simulink model "Model_tank"  (R2021b)
settings: Solver=ode45  StartTime=0.0  StopTime=80  RelTol=1e-3  EnableMultiTasking=on
values from neighbouring files (symbols this model uses):
  alpha1 = x1_val(2)    [Zbiorniki.m]    (also in c_table.mat = 0.278702458398; x0_table.mat = 0.278702458398)
  alpha2 = x2_val(2)    [Zbiorniki.m]    (also in c_table.mat = 0.328939614245; x0_table.mat = 0.328939614245)
  alpha3 = x3_val(2)    [Zbiorniki.m]    (also in c_table.mat = 0.404471667446; x0_table.mat = 0.404471667446)
  c1 = x1_val(1)    [Zbiorniki.m]    (also in c_table.mat = 41.0862215805; parametry.mat = 44.608; x0_table.mat = 41.0862215805)
  c2 = x2_val(1)    [Zbiorniki.m]    (also in c_table.mat = 36.7397635112; parametry.mat = 38.7996; x0_table.mat = 36.7397635112)
  c3 = x3_val(1)    [Zbiorniki.m]    (also in c_table.mat = 25.9394235455; parametry.mat = 39.9059; x0_table.mat = 25.9394235455)
undefined symbols (not defined in the file or in its folder): Set_Value_Motor
settings Model: Creator=Student  LastModifiedBy=Dawid
settings SolverCC: AlgebraicLoopSolver=TrustRegion
settings DataIOCC: LimitDataPoints=on  SaveFormat=Array  ReturnWorkspaceOutputs=off
settings OptimizationCC: LifeSpan=inf
settings DebuggingCC: SFUnexpectedBacktrackingDiag=warning  SFNoUnconditionalDefaultTransitionDiag=warning  SFExecutionAtInitializationDiag=none  SFMachineParentedDataDiag=warning  ArithmeticOperatorsInVariantConditions=warning
settings HardwareCC: ProdBitPerPointer=32  ProdBitPerSizeT=32  ProdBitPerPtrDiffT=32  ProdLargestAtomicFloat=None  ProdIntDivRoundTo=Undefined  ProdEndianess=Unspecified  ProdWordSize=32  ProdHWDeviceType=32-bit Generic
settings ModelReferenceCC: PropagateSignalLabelsOutOfModel=off
settings SFSimCC: SimUseLocalCustomCode=off  CustomCodeUndefinedFunction=UseInterfaceOnly
settings RTWCC: RTWUseLocalCustomCode=off
settings CodeAppCC: StateflowObjectComments=on
settings GRTTargetCC: TargetLangStandard=C89/C90 (ANSI)
settings ConfigComp: CovMetricSettings=dw  CovSaveCumulativeToWorkspaceVar=on  CovSaveSingleToWorkspaceVar=on  CovExternalEMLEnable=off

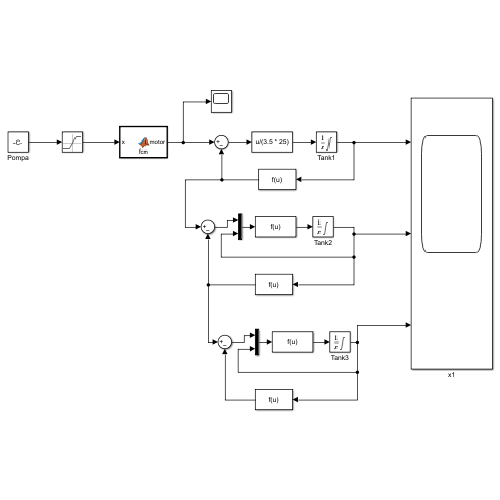
[thumbnail: Simulink's stored preview of the top-level diagram]
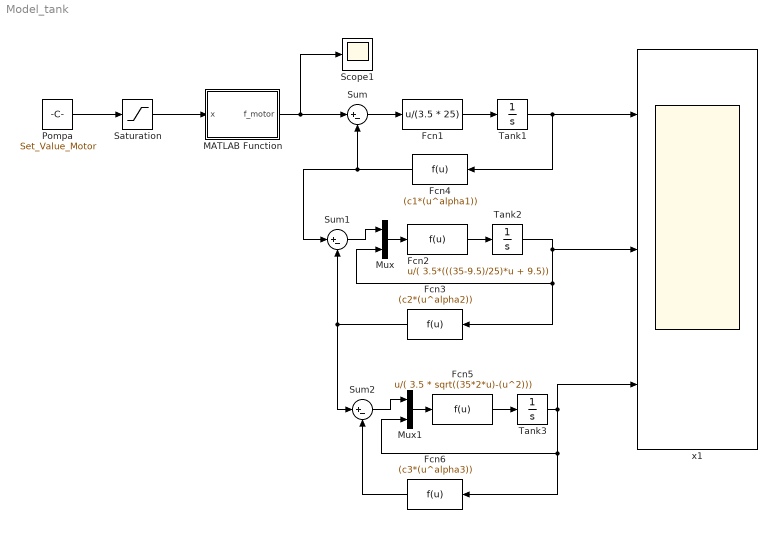
== system Model_tank ==
  Fcn1 : Fcn  Expr=u/(3.5 * 25)
  Fcn2 : Fcn  Expr=u/( 3.5*(((35-9.5)/25)*u + 9.5))
  Fcn3 : Fcn  Expr=(c2*(u^alpha2))
  Fcn4 : Fcn  Expr=(c1*(u^alpha1))
  Fcn5 : Fcn  Expr=u/( 3.5 * sqrt((35*2*u)-(u^2)))
  Fcn6 : Fcn  Expr=(c3*(u^alpha3))
  MATLAB Function : MATLAB Function  TreatAsAtomicUnit=on
  Mux : Mux  Inputs=2
  Mux1 : Mux  Inputs=2
  Pompa : Constant  Value=Set_Value_Motor
  Saturation : Saturate  UpperLimit=1  LowerLimit=0.5
  Scope1 : Scope
  Sum : Sum  Inputs=|+-
  Sum1 : Sum  Inputs=|+-
  Sum2 : Sum  Inputs=|+-
  Tank1 : Integrator  InitialCondition=0.01  LimitOutput=on  LowerSaturationLimit=0  ContinuousStateAttributes="\"Tank1\""
  Tank2 : Integrator  InitialCondition=0.01  LimitOutput=on  LowerSaturationLimit=0
  Tank3 : Integrator  InitialCondition=0.01  LimitOutput=on  LowerSaturationLimit=0
  x1 : Scope  NumInputPorts=3
  wires:
  Saturation/1 -> MATLAB Function/1(x)
  Pompa/1 -> Saturation/1
  MATLAB Function/1(f_motor) -> Scope1/1, Sum/1
  Sum/1 -> Fcn1/1
  Fcn1/1 -> Tank1/1
  Tank1/1 -> Fcn4/1, x1/1
  Fcn4/1 -> Sum1/1, Sum/2
  Fcn2/1 -> Tank2/1
  Tank2/1 -> Fcn3/1, Mux/2, x1/2
  Fcn3/1 -> Sum2/1, Sum1/2
  Mux/1 -> Fcn2/1
  Sum1/1 -> Mux/1
  Fcn6/1 -> Sum2/2
  Mux1/1 -> Fcn5/1
  Fcn5/1 -> Tank3/1
  Sum2/1 -> Mux1/1
  Tank3/1 -> x1/3, Mux1/2, Fcn6/1

== matlab function Model_tank/MATLAB Function ==
  data: x input; f_motor output
function f_motor = fcn(x)

a1_motor = 4.336406289988628e+02;
a2_motor = -1.346640151767827e+03;
a3_motor = 1.555231837686545e+03;
a4_motor = -5.004734794411548e+02;

f_motor = a1_motor * x^3 + a2_motor * x^2 + a3_motor * x + a4_motor;
